simulink model "LineTrace_2025a"  (R2025a)
settings: Solver=FixedStepAuto  StartTime=0  StopTime=10  FixedStep=0.001  RelTol=1e-3
undefined symbols (not defined in the file): Rec, SDTV, Sim3dSensor
libraries: visionsinks x9, sim3dcameralib x9, sim3dlib x4, visionconversions x4
settings Model: ModifiedByFormat=The MathWorks, Inc.  Creator=The MathWorks, Inc.  LastModifiedBy=The MathWorks, Inc.
settings DataIOCC: SaveFormat=StructureWithTime
settings OptimizationCC: BlockReduction=off  BufferReuse=off
settings DebuggingCC: AlgebraicLoopMsg=none  SubsystemReferenceDiagnosticForUnitTest=warning
settings RTWCC: GPUComputeCapability=3.5

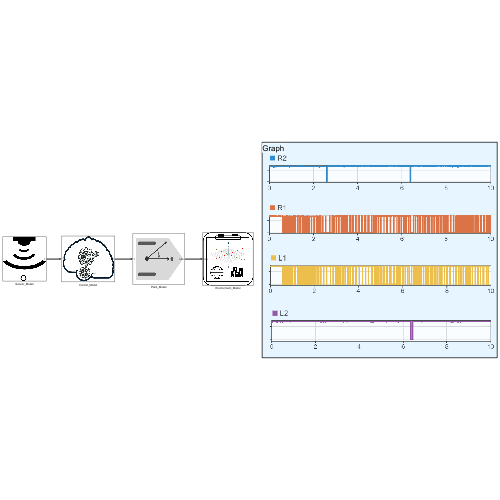
[thumbnail: Simulink's stored preview of the top-level diagram]
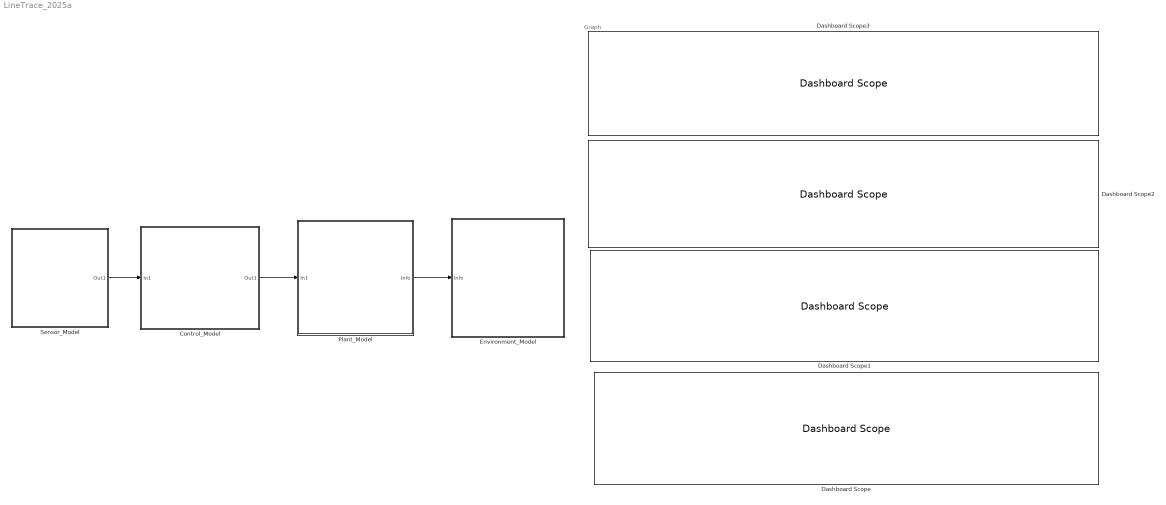
== system LineTrace_2025a ==
  note: Graph
  Control_Model : Subsystem
      mask Display: image('Control.png');
  Dashboard Scope{,1..3} (4 alike) : DashboardScope  Ymin=0  Ymax=3200  FontColor=[0.0, 0.0, 0.0]
      settings: TickLabels=T-Axis
  Environment_Model : Subsystem
      mask Display: image('Environment.png');
  Plant_Model : Subsystem
      mask Display: image('Plant.png');
  Sensor_Model : Subsystem
      mask Display: image('Sensor.png');
  wires:
  Sensor_Model/1(Out1) -> Control_Model/1(In1)
  Control_Model/1(Out1) -> Plant_Model/1(In1)
  Plant_Model/1(Info) -> Environment_Model/1(Info)

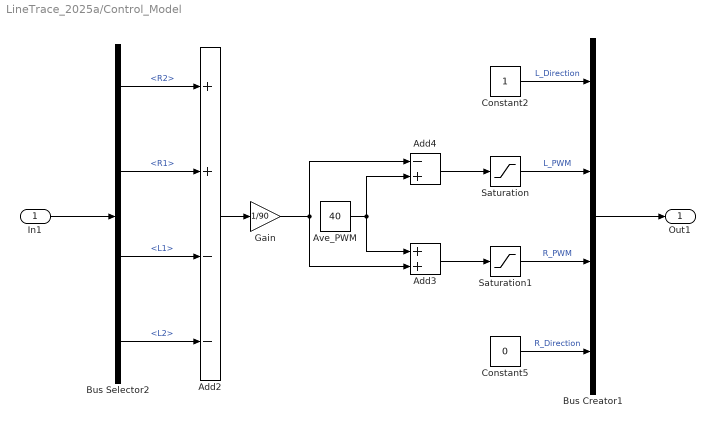
== system LineTrace_2025a/Control_Model ==
  In1 : Inport
  Add2 : Sum  Inputs=++--  OutDataTypeStr=double
  Add3 : Sum
  Add4 : Sum  Inputs=-+
  Ave_PWM : Constant  Value=40
  Bus Creator1 : BusCreator  Inputs=4
  Bus Selector2 : BusSelector  OutputSignals=R2,R1,L1,L2
  Constant2 : Constant
  Constant5 : Constant  Value=0
  Gain : Gain  Gain=1/90
  Saturation : Saturate  UpperLimit=99  LowerLimit=0
  Saturation1 : Saturate  UpperLimit=99  LowerLimit=0
  Out1 : Outport
  wires:
  Bus Selector2/2 -> Add2/2  "<R1>"
  In1/1 -> Bus Selector2/1
  Ave_PWM/1 -> Add4/2, Add3/1
  Add2/1 -> Gain/1
  Bus Selector2/4 -> Add2/4  "<L2>"
  Saturation1/1 -> Bus Creator1/3  "R_PWM"
  Saturation/1 -> Bus Creator1/2  "L_PWM"
  Constant5/1 -> Bus Creator1/4  "R_Direction"
  Add4/1 -> Saturation/1
  Add3/1 -> Saturation1/1
  Bus Selector2/1 -> Add2/1  "<R2>"
  Bus Selector2/3 -> Add2/3  "<L1>"
  Constant2/1 -> Bus Creator1/1  "L_Direction"
  Bus Creator1/1 -> Out1/1
  Gain/1 -> Add4/1, Add3/2

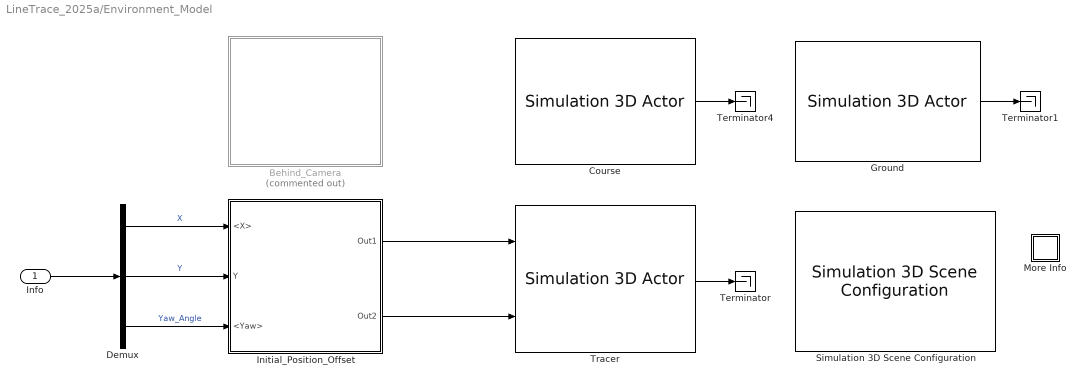
== system LineTrace_2025a/Environment_Model ==
  Info : Inport
  Behind_Camera : Subsystem  Commented=on  mask{R2_X=-0.7, R2_Y=0, R2_Z=0.2, R2_Rot_X=0, R2_Rot_Y=-pi/6, R2_Rot_Z=0}
      mask prompts: R2_X "Initial Sensor Position (X) [m]"; R2_Y "Initial Sensor Position (Y) [m]"; R2_Z "Initial Sensor Position (Z) [m]"; R2_Rot_X "Rotation Offset (X):  Roll [rad]"; R2_Rot_Y "Rotation Offset (Y): Pitch[rad]"; R2_Rot_Z "Rotation Offset (Z):  Yaw [rad]"
      mask help:
      | This block sets the initial position (X, Y, Z) and orientation (Roll, Pitch, Yaw) of the robot.
      | Simply enter the parameters to adjust accordingly.
      mask DialogControl DescTextVar Prompt: This block sets the initial position (X, Y, Z) and orientation (Roll, Pitch, Yaw) of a sensor. Simply enter the parameters to adjust accordingly. Since the sensor is facing directly downward, the initial value of Pitch is set to 90 degrees.
      mask Display: image('スクリーンショット 2025-03-12 191128.png');
  Course : sim3dlib/Simulation 3D Actor  ActorName=Course  ParentName=Scene Origin  Operation=Create at setup  InitScriptText=|  SampleTime=-1  Translation=single([0 0 0])  Rotation=single([0 0 0])  Scale=0.01*[1 1 0.01]  aMode=5  ActorTag=Course  ActorType=Sim3dActor  ID=C
      | Actor.PreciseContacts = true;
      | Actor.Physics = true;
      | Actor.Color = [0 0 0];
      | actor.Shininess = 0;
      | actor.Metallic = 0;
      settings: LibrarySourceBlock=sl3dlib/Simulation 3D/Simulation 3D Actor
  Demux : Demux  Outputs=3
  Ground : sim3dlib/Simulation 3D Actor  ActorName=Ground  ParentName=Scene Origin  Operation=Create at setup  InitScriptText=|  SampleTime=-1  Translation=single([0 0 0])  Rotation=single([0 0 0])  Scale=single([1 1 1])  aMode=5  ActorTag=Ground  ActorType=Sim3dActor  ID=C
      | Actor.createShape('plane', [3 3 0.001]);
      | Actor.PreciseContacts = true;
      | Actor.Physics = true;
      | Actor.Color = [1 1 1];
      | actor.Shininess = 0;
      | actor.Metallic = 0;
      settings: LibrarySourceBlock=sl3dlib/Simulation 3D/Simulation 3D Actor
  Initial_Position_Offset : Subsystem  mask{Offset_X=0, Offset_Y=0, Offset_Z=0, Offset_Rot_X=0, Offset_Rot_Y=0, Offset_Rot_Z=0}
      mask prompts: Offset_X "Translation Offset (X) [m]"; Offset_Y "Translation Offset (Y) [m]"; Offset_Z "Translation Offset (Z) [m]"; Offset_Rot_X "Rotation Offset (X):  Roll [rad]"; Offset_Rot_Y "Rotation Offset (Y): Pitch[rad]"; Offset_Rot_Z "Rotation Offset (Z):  Yaw [rad]"
      mask DialogControl DescTextVar Prompt: This block sets the initial position (X, Y, Z) and orientation (Roll, Pitch, Yaw) of the robot. Simply enter the parameters to adjust accordingly.
      mask Display: image('画像2.png');
  More Info : Subsystem
      settings: OpenFcn=showExample('sl3d/CreateActorSTLFileExample')
      mask Display: disp('?')
  Simulation 3D Scene Configuration : sim3dlib/Simulation 3D Scene Configuration  Priority=0  ProjectFormat=Default Scenes  SceneDesc=Empty scene  ProjectName=C:\Program Files\MATLAB\R2025a\toolbox\shared\sim3d_projects\automotive_project_windows\UE\WindowsNoEditor\VehicleSimulation.exe  ScenePath=/Game/Maps/HwStrght  EnableOpenDRIVE=off  vehTagList={'Course';'Custom';'Ground';'Scene Origin';'Tracer'}  vehTag=Custom  AttachedCameraRelativeTranslation=[0 0 0]  FreeCameraDefaultInitialTranslation=[-6, 0, 2]  AttachedCameraRelativeRotation=[0 0 0]  FreeCameraDefaultInitialRotation=[0, -15, 0]  ViewpointName=Custom  FreeCameraInitialTranslation=[0 0.6 1.5]  ViewpointTranslation=[0 0.6 1.5]  FreeCameraInitialRotation=[0 -90 90]  ViewpointRotation=[0 -90 90]  OpVisEn=off  Ts=.01  EnableWindow=on  EnableRemoteAccess=off  EnableWeather=off  SunAzimuth=90  SunAltitude=40.0  EnableGeospatialSun=off  Latitude=0  Longitude=0  Date=2023-01-01  Time=10:30:00  GeoTimeZone=-5.0  SunDaylightSaving=off  wind=1  clouds=10  EnableVolumetricClouds=off  CloudCoverage=0  CloudAltitude=6  fog=0  rain=0  RaindropsEffect=off  SnowDensity=0  EnableGeospatial=off  TilesetSource=Earth terrain  UseTrueOrigin=off  OriginHeight=200  OriginLatitude=40.744652  OriginLongitude=-73.988864  MapStyle=Aerial  AdditionalAssetIDs=[]  UseAdvancedSunSky=off  SolarTime=11  TimeZone=-5  Day=21  Month=9  Year=2022  UseDaylightSavingTime=on  DSTStartDay=10  DSTStartMonth=3  DSTEndDay=3  DSTEndMonth=11  DSTSwitchHour=2  sensorTag=MainCamera2  sensorId=2  sensorName=MainCamera2  mountLoc=Origin  offsetFlag=off  tmountOffset=[0, 0, 0]  rmountOffset=[0, 0, 0]  HorizontalResolution=1280  VerticalResolution=720  HorizontalFOV=60  mountPoint=[0 0 0]  mountOrientation=[0 0 0]  aMode=5  ID=2  GeoTrigger=Inactive  ViewNameList={'Custom'}  ViewTranslationList={'[0 0.6 1.5]'}  ViewRotationList={'[0 -90 90]'}
      settings: LibrarySourceBlock=sl3dlib/Simulation 3D/Environment/Simulation 3D Scene Configuration
  Terminator : Terminator
  Terminator1 : Terminator
  Terminator4 : Terminator
  Tracer : sim3dlib/Simulation 3D Actor  Priority=1  ActorName=Tracer  ParentName=Scene Origin  Operation=Create at setup  InitScriptText=|  SampleTime=-1  Translation=[0 0 0]  Rotation=[0 0 0]  Scale=0.01*[1 1 1]  InputsText=Tracer.Translation Tracer.Rotation  aMode=5  ActorTag=Tracer  ActorType=Sim3dActor  ID=C
      | Actor.Shadows = true;
      | Actor.Color = [0 0 0];
  wires:
  Course/1 -> Terminator4/1
  Ground/1 -> Terminator1/1
  Tracer/1 -> Terminator/1
  Initial_Position_Offset/2(Out2) -> Tracer/2
  Info/1 -> Demux/1
  Demux/1 -> Initial_Position_Offset/1(<X>)  "X"
  Demux/2 -> Initial_Position_Offset/2(Y)  "Y"
  Demux/3 -> Initial_Position_Offset/3(<Yaw>)  "Yaw_Angle"
  Initial_Position_Offset/1(Out1) -> Tracer/1

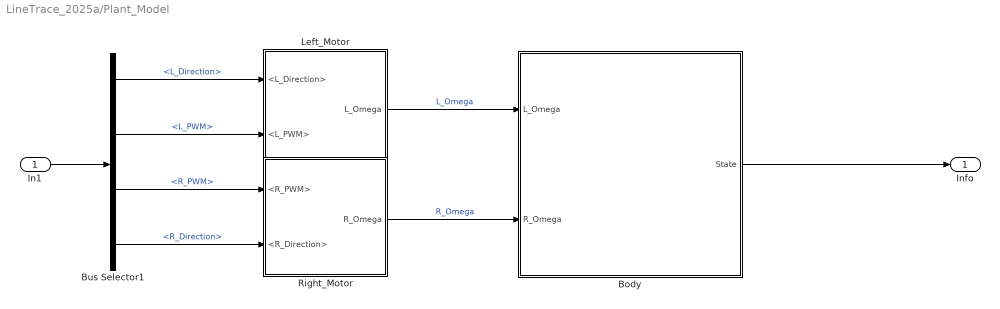
== system LineTrace_2025a/Plant_Model ==
  In1 : Inport
  Body : Subsystem  mask{Diameter_L=0.0205, Diameter_R=0.0205, Tread=0.085}
      mask prompts: Diameter_L "Left Wheel Diameter [m]"; Diameter_R "Right Wheel Diameter [m]"; Tread "Track Width [m]"
      mask DialogControl DescGroupVar Prompt: Differential Drive Kinematic Model
      mask DialogControl DescTextVar Prompt: Compute vehicle motion using a differential drive kinematic model.   The block inputs are two scalar values that depend on the value of the Vehicle inputs parameter and can either accept left and right wheel speeds, or vehicle speed and heading angular velocity. The block outputs a three-element state vector of xy-positions and vehicle heading, [x y theta], and their time derivatives, stateDot.
      mask Display: image('スクリーンショット 2025-02-13 142952.png');
  Bus Selector1 : BusSelector  OutputSignals=L_Direction,L_PWM,R_PWM,R_Direction
  Left_Motor : Subsystem
      mask Display: image('L_Motor.png');
  Right_Motor : Subsystem
      mask Display: image('R_Motor.png');
  Info : Outport
  wires:
  Body/1(State) -> Info/1
  In1/1 -> Bus Selector1/1
  Bus Selector1/1 -> Left_Motor/1(<L_Direction>)  "<L_Direction>"
  Bus Selector1/2 -> Left_Motor/2(<L_PWM>)  "<L_PWM>"
  Left_Motor/1(L_Omega) -> Body/1(L_Omega)  "L_Omega"
  Bus Selector1/3 -> Right_Motor/1(<R_PWM>)  "<R_PWM>"
  Bus Selector1/4 -> Right_Motor/2(<R_Direction>)  "<R_Direction>"
  Right_Motor/1(R_Omega) -> Body/2(R_Omega)  "R_Omega"

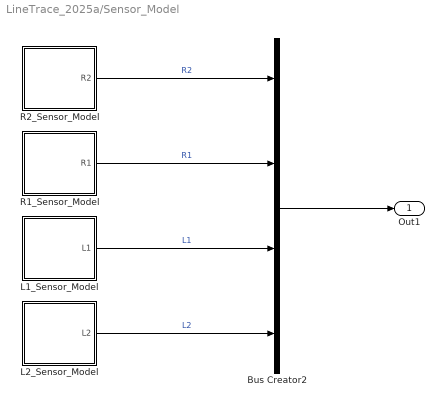
== system LineTrace_2025a/Sensor_Model ==
  Bus Creator2 : BusCreator  Inputs=4
  L1_Sensor_Model : Subsystem  mask{L1_X=0.0675, L1_Y=0.0115, L1_Z=0.0145, L1_Rot_X=0, L1_Rot_Y=-pi/2, L1_Rot_Z=0}
      mask prompts: L1_X "Initial Sensor Position (X) [m]"; L1_Y "Initial Sensor Position (Y) [m]"; L1_Z "Initial Sensor Position (Z) [m]"; L1_Rot_X "Rotation Offset (X):  Roll [rad]"; L1_Rot_Y "Rotation Offset (Y): Pitch[rad]"; L1_Rot_Z "Rotation Offset (Z):  Yaw [rad]"
      mask DialogControl DescTextVar Prompt: This block sets the initial position (X, Y, Z) and orientation (Roll, Pitch, Yaw) of a sensor. Simply enter the parameters to adjust accordingly. Since the sensor is facing directly downward, the initial value of Pitch is set to 90 degrees.
      mask Display: image('L1.png');
  L2_Sensor_Model : Subsystem  mask{L2_X=0.075, L2_Y=0.0325, L2_Z=0.0145, L2_Rot_X=0, L2_Rot_Y=-pi/2, L2_Rot_Z=0}
      mask prompts: L2_X "Initial Sensor Position (X) [m]"; L2_Y "Initial Sensor Position (Y) [m]"; L2_Z "Initial Sensor Position (Z) [m]"; L2_Rot_X "Rotation Offset (X):  Roll [rad]"; L2_Rot_Y "Rotation Offset (Y): Pitch[rad]"; L2_Rot_Z "Rotation Offset (Z):  Yaw [rad]"
      mask DialogControl DescTextVar Prompt: This block sets the initial position (X, Y, Z) and orientation (Roll, Pitch, Yaw) of a sensor. Simply enter the parameters to adjust accordingly. Since the sensor is facing directly downward, the initial value of Pitch is set to 90 degrees.
      mask Display: image('L2.png');
  R1_Sensor_Model : Subsystem  mask{R1_X=0.0675, R1_Y=-0.0115, R1_Z=0.0145, R1_Rot_X=0, R1_Rot_Y=-pi/2, R1_Rot_Z=0}
      mask prompts: R1_X "Initial Sensor Position (X) [m]"; R1_Y "Initial Sensor Position (Y) [m]"; R1_Z "Initial Sensor Position (Z) [m]"; R1_Rot_X "Rotation Offset (X):  Roll [rad]"; R1_Rot_Y "Rotation Offset (Y): Pitch[rad]"; R1_Rot_Z "Rotation Offset (Z):  Yaw [rad]"
      mask DialogControl DescTextVar Prompt: This block sets the initial position (X, Y, Z) and orientation (Roll, Pitch, Yaw) of a sensor. Simply enter the parameters to adjust accordingly. Since the sensor is facing directly downward, the initial value of Pitch is set to 90 degrees.
      mask Display: image('R1.png');
  R2_Sensor_Model : Subsystem  mask{R2_X=0.075, R2_Y=-0.0325, R2_Z=0.0145, R2_Rot_X=0, R2_Rot_Y=-pi/2, R2_Rot_Z=0}
      mask prompts: R2_X "Initial Sensor Position (X) [m]"; R2_Y "Initial Sensor Position (Y) [m]"; R2_Z "Initial Sensor Position (Z) [m]"; R2_Rot_X "Rotation Offset (X):  Roll [rad]"; R2_Rot_Y "Rotation Offset (Y): Pitch[rad]"; R2_Rot_Z "Rotation Offset (Z):  Yaw [rad]"
      mask help:
      | This block sets the initial position (X, Y, Z) and orientation (Roll, Pitch, Yaw) of the robot.
      | Simply enter the parameters to adjust accordingly.
      mask DialogControl DescTextVar Prompt: This block sets the initial position (X, Y, Z) and orientation (Roll, Pitch, Yaw) of a sensor. Simply enter the parameters to adjust accordingly. Since the sensor is facing directly downward, the initial value of Pitch is set to 90 degrees.
      mask Display: image('R2.png');
  Out1 : Outport
  wires:
  R1_Sensor_Model/1(R1) -> Bus Creator2/2  "R1"
  L1_Sensor_Model/1(L1) -> Bus Creator2/3  "L1"
  R2_Sensor_Model/1(R2) -> Bus Creator2/1  "R2"
  L2_Sensor_Model/1(L2) -> Bus Creator2/4  "L2"
  Bus Creator2/1 -> Out1/1

== system LineTrace_2025a/Environment_Model/Behind_Camera ==
  Back Camera : Subsystem
      mask Display: image('スクリーンショット 2025-03-18 120217.png');

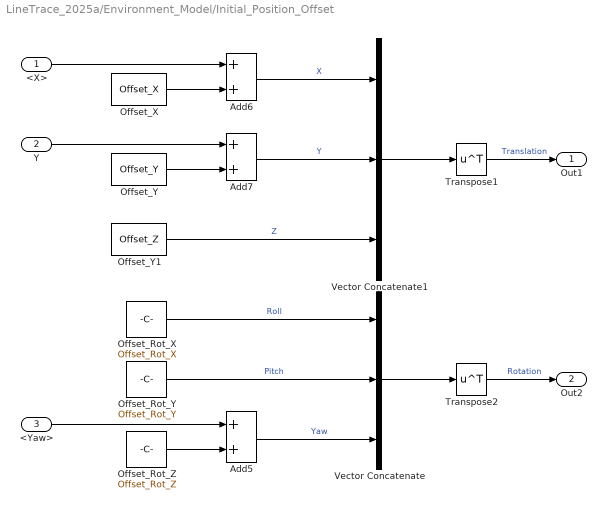
== system LineTrace_2025a/Environment_Model/Initial_Position_Offset ==
  <X> : Inport
  Y : Inport  Port=2
  <Yaw> : Inport  Port=3
  Add5 : Sum
  Add6 : Sum
  Add7 : Sum
  Offset_Rot_X : Constant  Value=Offset_Rot_X
  Offset_Rot_Y : Constant  Value=Offset_Rot_Y
  Offset_Rot_Z : Constant  Value=Offset_Rot_Z
  Offset_X : Constant  Value=Offset_X
  Offset_Y : Constant  Value=Offset_Y
  Offset_Y1 : Constant  Value=Offset_Z
  Transpose1 : Math  Operator=transpose
  Transpose2 : Math  Operator=transpose
  Vector Concatenate : Concatenate  NumInputs=3
  Vector Concatenate1 : Concatenate  NumInputs=3
  Out1 : Outport
  Out2 : Outport  Port=2
  wires:
  Add5/1 -> Vector Concatenate/3  "Yaw"
  Offset_Rot_X/1 -> Vector Concatenate/1  "Roll"
  Add7/1 -> Vector Concatenate1/2  "Y"
  Offset_Y1/1 -> Vector Concatenate1/3  "Z"
  Add6/1 -> Vector Concatenate1/1  "X"
  Offset_X/1 -> Add6/2
  Offset_Rot_Z/1 -> Add5/2
  Offset_Y/1 -> Add7/2
  Offset_Rot_Y/1 -> Vector Concatenate/2  "Pitch"
  Vector Concatenate/1 -> Transpose2/1
  Transpose1/1 -> Out1/1  "Translation"
  <Yaw>/1 -> Add5/1
  Y/1 -> Add7/1
  Vector Concatenate1/1 -> Transpose1/1
  Transpose2/1 -> Out2/1  "Rotation"
  <X>/1 -> Add6/1

== system LineTrace_2025a/Environment_Model/More Info ==

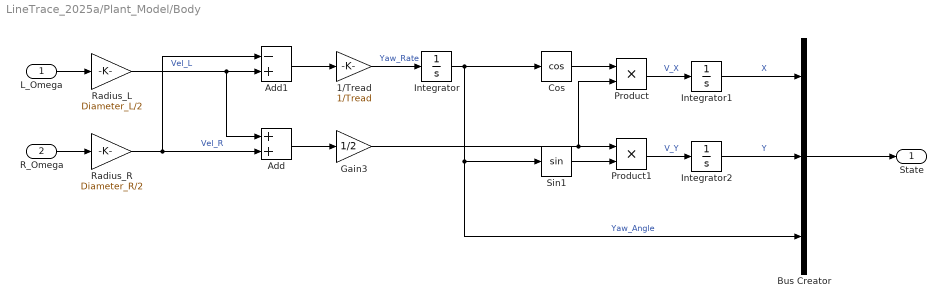
== system LineTrace_2025a/Plant_Model/Body ==
  L_Omega : Inport
  R_Omega : Inport  Port=2
  1/Tread : Gain  Gain=1/Tread
  Add : Sum
  Add1 : Sum  Inputs=-+
  Bus Creator : BusCreator  Inputs=3
  Cos : Trigonometry  Operator=cos
  Gain3 : Gain  Gain=1/2
  Integrator : Integrator
  Integrator1 : Integrator
  Integrator2 : Integrator
  Product : Product
  Product1 : Product
  Radius_L : Gain  Gain=Diameter_L/2
  Radius_R : Gain  Gain=Diameter_R/2
  Sin1 : Trigonometry
  State : Outport
  wires:
  Integrator/1 -> Bus Creator/3, Sin1/1, Cos/1  "Yaw_Angle"
  Product/1 -> Integrator1/1  "V_X"
  1/Tread/1 -> Integrator/1  "Yaw_Rate"
  Add/1 -> Gain3/1
  Sin1/1 -> Product1/2
  Cos/1 -> Product/1
  L_Omega/1 -> Radius_L/1
  Gain3/1 -> Product/2, Product1/1
  Product1/1 -> Integrator2/1  "V_Y"
  Integrator1/1 -> Bus Creator/1  "X"
  Add1/1 -> 1/Tread/1
  R_Omega/1 -> Radius_R/1
  Integrator2/1 -> Bus Creator/2  "Y"
  Bus Creator/1 -> State/1
  Radius_L/1 -> Add/1, Add1/2  "Vel_L"
  Radius_R/1 -> Add/2, Add1/1  "Vel_R"

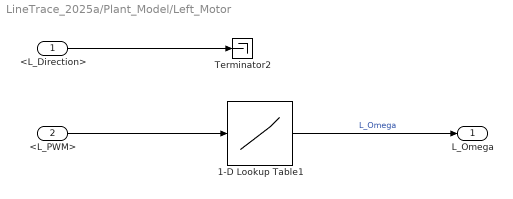
== system LineTrace_2025a/Plant_Model/Left_Motor ==
  <L_Direction> : Inport
  <L_PWM> : Inport  Port=2
  1-D Lookup Table1 : Lookup_n-D  NumberOfTableDimensions=1  BreakpointsForDimension1=[-100:20:100]  Table=tanh([-5:5])*50  InternalRulePriority=Speed  RndMeth=Simplest
  Terminator2 : Terminator
  L_Omega : Outport
  wires:
  1-D Lookup Table1/1 -> L_Omega/1  "L_Omega"
  <L_Direction>/1 -> Terminator2/1
  <L_PWM>/1 -> 1-D Lookup Table1/1

== system LineTrace_2025a/Plant_Model/Right_Motor ==
  <R_PWM> : Inport
  <R_Direction> : Inport  Port=2
  1-D Lookup Table1 : Lookup_n-D  NumberOfTableDimensions=1  BreakpointsForDimension1=[-100:20:100]  Table=tanh([-5:5])*50  InternalRulePriority=Speed  RndMeth=Simplest
  Terminator3 : Terminator
  R_Omega : Outport
  wires:
  <R_PWM>/1 -> 1-D Lookup Table1/1
  1-D Lookup Table1/1 -> R_Omega/1  "R_Omega"
  <R_Direction>/1 -> Terminator3/1

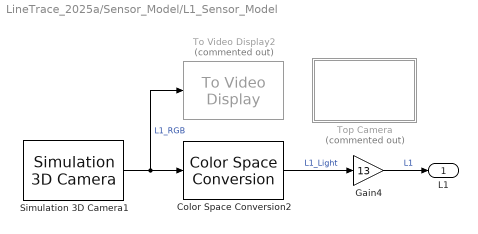
== system LineTrace_2025a/Sensor_Model/L1_Sensor_Model ==
  Color Space Conversion2 : visionconversions/Color Space  Conversion  conversion=Obsolete  conversionActive=R'G'B' to intensity  wp_str=D65  rec=Rec. 601 (SDTV)  sys=1125/60/2:1  imagePorts=One multidimensional signal
  Gain4 : Gain  Gain=13
  Simulation 3D Camera1 : sim3dcameralib/Simulation 3D Camera  Priority=1  sensorTag=Sim3dSensor$  sensorId=36  sensorName=Sim3dSensor$  vehTagList={'Course';'Ground';'Scene Origin';'Tracer'}  vehTag=Tracer  CoordinateSystem=Default  mountLoc=Origin  offsetFlag=on  tmountOffset=100*[L1_X, -L1_Y, L1_Z+0.089]  extTmount=off  rmountOffset=[L1_Rot_X L1_Rot_Y L1_Rot_Z]  extRmount=off  FocalLength=[75000 75000]  OpticalCenter=[0.5 0.5]  ImageSize=[1 1]  RadialDistortion=[0, 0]  TangentialDistortion=[0, 0]  SensorSkew=0  VisualizeFieldOfView=off  FieldOfViewRange=61  DepthOutportEnabled=off  SemanticOutportEnabled=off  TransformOutportEnabled=off  SampleTime=-1  mountPoint=[6.75 -1.15 10.35]  mountOrientation=[0 -1.5707963267949 0]  aMode=5  ID=36
      settings: LibrarySourceBlock=Simulation 3D Camera
  To Video Display2 : visionsinks/To Video Display  Commented=on  windowSizeMode=Normal  openAtMdlStart=on  fullScreen=off  videoWindowX=536805376  videoWindowY=536805376  saveWindowSize=off  videoWindowWidth=956  videoWindowHeight=1146  inputColorFormat=RGB  inputType=Obsolete  imagePorts=One multidimensional signal  OutputDevice=On-screen video monitor  dataOrg=Column-major  isWindowOpen=off
  Top Camera : Subsystem  Commented=on
      mask Display: image('スクリーンショット 2025-03-18 120217.png');
  L1 : Outport
  wires:
  Simulation 3D Camera1/1 -> To Video Display2/1, Color Space Conversion2/1  "L1_RGB"
  Gain4/1 -> L1/1  "L1"
  Color Space Conversion2/1 -> Gain4/1  "L1_Light"

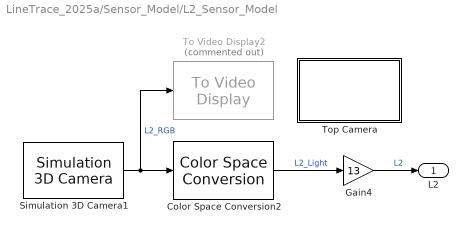
== system LineTrace_2025a/Sensor_Model/L2_Sensor_Model ==
  Color Space Conversion2 : visionconversions/Color Space  Conversion  conversion=Obsolete  conversionActive=R'G'B' to intensity  wp_str=D65  rec=Rec. 601 (SDTV)  sys=1125/60/2:1  imagePorts=One multidimensional signal
  Gain4 : Gain  Gain=13
  Simulation 3D Camera1 : sim3dcameralib/Simulation 3D Camera  Priority=1  sensorTag=Sim3dSensor&  sensorId=38  sensorName=Sim3dSensor&  vehTagList={'Course';'Ground';'Scene Origin';'Tracer'}  vehTag=Tracer  CoordinateSystem=Default  mountLoc=Origin  offsetFlag=on  tmountOffset=100*[L2_X, -L2_Y, L2_Z+0.089]  extTmount=off  rmountOffset=[L2_Rot_X L2_Rot_Y L2_Rot_Z]  extRmount=off  FocalLength=[75000 75000]  OpticalCenter=[0.5 0.5]  ImageSize=[1 1]  RadialDistortion=[0, 0]  TangentialDistortion=[0, 0]  SensorSkew=0  VisualizeFieldOfView=off  FieldOfViewRange=61  DepthOutportEnabled=off  SemanticOutportEnabled=off  TransformOutportEnabled=off  SampleTime=-1  mountPoint=[7.5 -3.25 10.35]  mountOrientation=[0 -1.5707963267949 0]  aMode=5  ID=38
      settings: LibrarySourceBlock=Simulation 3D Camera
  To Video Display2 : visionsinks/To Video Display  Commented=on  windowSizeMode=Normal  openAtMdlStart=on  fullScreen=off  videoWindowX=536805376  videoWindowY=536805376  saveWindowSize=off  videoWindowWidth=956  videoWindowHeight=1146  inputColorFormat=RGB  inputType=Obsolete  imagePorts=One multidimensional signal  OutputDevice=On-screen video monitor  dataOrg=Column-major  isWindowOpen=off
  Top Camera : Subsystem
      mask Display: image('スクリーンショット 2025-03-18 120217.png');
  L2 : Outport
  wires:
  Color Space Conversion2/1 -> Gain4/1  "L2_Light"
  Simulation 3D Camera1/1 -> To Video Display2/1, Color Space Conversion2/1  "L2_RGB"
  Gain4/1 -> L2/1  "L2"

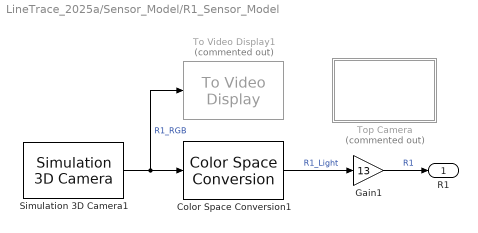
== system LineTrace_2025a/Sensor_Model/R1_Sensor_Model ==
  Color Space Conversion1 : visionconversions/Color Space  Conversion  conversion=Obsolete  conversionActive=R'G'B' to intensity  wp_str=D65  rec=Rec. 601 (SDTV)  sys=1125/60/2:1  imagePorts=One multidimensional signal
  Gain1 : Gain  Gain=13
  Simulation 3D Camera1 : sim3dcameralib/Simulation 3D Camera  Priority=1  sensorTag="Sim3dSensor\""  sensorId=34  sensorName="Sim3dSensor\""  vehTagList={'Course';'Ground';'Scene Origin';'Tracer'}  vehTag=Tracer  CoordinateSystem=Default  mountLoc=Origin  offsetFlag=on  tmountOffset=100*[R1_X, -R1_Y, R1_Z+0.089]  extTmount=off  rmountOffset=[R1_Rot_X R1_Rot_Y R1_Rot_Z]  extRmount=off  FocalLength=[75000 75000]  OpticalCenter=[0.5 0.5]  ImageSize=[1 1]  RadialDistortion=[0, 0]  TangentialDistortion=[0, 0]  SensorSkew=0  VisualizeFieldOfView=off  FieldOfViewRange=61  DepthOutportEnabled=off  SemanticOutportEnabled=off  TransformOutportEnabled=off  SampleTime=-1  mountPoint=[6.75 1.15 10.35]  mountOrientation=[0 -1.5707963267949 0]  aMode=5  ID=34
      settings: LibrarySourceBlock=Simulation 3D Camera
  To Video Display1 : visionsinks/To Video Display  Commented=on  windowSizeMode=Normal  openAtMdlStart=on  fullScreen=off  videoWindowX=536805376  videoWindowY=536805376  saveWindowSize=off  videoWindowWidth=956  videoWindowHeight=1146  inputColorFormat=RGB  inputType=Obsolete  imagePorts=One multidimensional signal  OutputDevice=On-screen video monitor  dataOrg=Column-major  isWindowOpen=off
  Top Camera : Subsystem  Commented=on
      mask Display: image('スクリーンショット 2025-03-18 120217.png');
  R1 : Outport
  wires:
  Color Space Conversion1/1 -> Gain1/1  "R1_Light"
  Gain1/1 -> R1/1  "R1"
  Simulation 3D Camera1/1 -> Color Space Conversion1/1, To Video Display1/1  "R1_RGB"

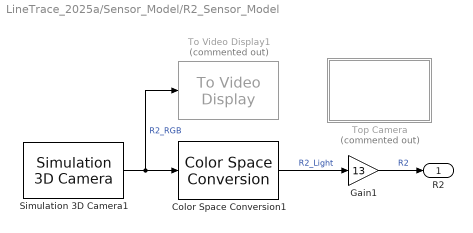
== system LineTrace_2025a/Sensor_Model/R2_Sensor_Model ==
  Color Space Conversion1 : visionconversions/Color Space  Conversion  conversion=Obsolete  conversionActive=R'G'B' to intensity  wp_str=D65  rec=Rec. 601 (SDTV)  sys=1125/60/2:1  imagePorts=One multidimensional signal
  Gain1 : Gain  Gain=13
  Simulation 3D Camera1 : sim3dcameralib/Simulation 3D Camera  Priority=1  sensorTag=Sim3dSensor  sensorId=32  sensorName=Sim3dSensor  vehTagList={'Course';'Ground';'Scene Origin';'Tracer'}  vehTag=Tracer  CoordinateSystem=Default  mountLoc=Origin  offsetFlag=on  tmountOffset=100*[R2_X, -R2_Y, R2_Z+0.089]  extTmount=off  rmountOffset=[R2_Rot_X R2_Rot_Y R2_Rot_Z]  extRmount=off  FocalLength=[75000 75000]  OpticalCenter=[0.5 0.5]  ImageSize=[1 1]  RadialDistortion=[0, 0]  TangentialDistortion=[0, 0]  SensorSkew=0  VisualizeFieldOfView=off  FieldOfViewRange=61  DepthOutportEnabled=off  SemanticOutportEnabled=off  TransformOutportEnabled=off  SampleTime=-1  mountPoint=[7.5 3.25 10.35]  mountOrientation=[0 -1.5707963267949 0]  aMode=5  ID=32
      settings: LibrarySourceBlock=Simulation 3D Camera
  To Video Display1 : visionsinks/To Video Display  Commented=on  windowSizeMode=Normal  openAtMdlStart=on  fullScreen=off  videoWindowX=536805376  videoWindowY=536805376  saveWindowSize=off  videoWindowWidth=956  videoWindowHeight=1146  inputColorFormat=RGB  inputType=Obsolete  imagePorts=One multidimensional signal  OutputDevice=On-screen video monitor  dataOrg=Column-major  isWindowOpen=off
  Top Camera : Subsystem  Commented=on
      mask Display: image('スクリーンショット 2025-03-18 120217.png');
  R2 : Outport
  wires:
  Gain1/1 -> R2/1  "R2"
  Color Space Conversion1/1 -> Gain1/1  "R2_Light"
  Simulation 3D Camera1/1 -> Color Space Conversion1/1, To Video Display1/1  "R2_RGB"

== system LineTrace_2025a/Environment_Model/Behind_Camera/Back Camera ==
  Behind_Camera : visionsinks/To Video Display  windowSizeMode=Normal  openAtMdlStart=on  fullScreen=off  videoWindowX=536805376  videoWindowY=536805376  saveWindowSize=off  videoWindowWidth=1920  videoWindowHeight=1076  inputColorFormat=RGB  inputType=Obsolete  imagePorts=One multidimensional signal  OutputDevice=On-screen video monitor  dataOrg=Column-major  isWindowOpen=off
  Simulation 3D Camera : sim3dcameralib/Simulation 3D Camera  Priority=1  sensorTag=Sim3dSensor(  sensorId=40  sensorName=Sim3dSensor(  vehTagList={'Course';'Ground';'Scene Origin';'Tracer'}  vehTag=Tracer  CoordinateSystem=Default  mountLoc=Origin  offsetFlag=on  tmountOffset=100*[R2_X, -R2_Y, R2_Z+0.3]  extTmount=off  rmountOffset=[R2_Rot_X R2_Rot_Y R2_Rot_Z]  extRmount=off  FocalLength=[2000 2000]  OpticalCenter=[500 500]  ImageSize=[1000 1000]  RadialDistortion=[0, 0]  TangentialDistortion=[0, 0]  SensorSkew=0  VisualizeFieldOfView=off  FieldOfViewRange=61  DepthOutportEnabled=off  SemanticOutportEnabled=off  TransformOutportEnabled=off  SampleTime=-1  mountPoint=[-70 0 50]  mountOrientation=[0 -0.523598775598299 0]  aMode=5  ID=40
      settings: LibrarySourceBlock=Simulation 3D Camera
  wires:
  Simulation 3D Camera/1 -> Behind_Camera/1

== system LineTrace_2025a/Sensor_Model/L1_Sensor_Model/Top Camera ==
  L1_Camera : visionsinks/To Video Display  windowSizeMode=Normal  openAtMdlStart=on  fullScreen=off  videoWindowX=536805376  videoWindowY=536805376  saveWindowSize=off  videoWindowWidth=1894  videoWindowHeight=1134  inputColorFormat=RGB  inputType=Obsolete  imagePorts=One multidimensional signal  OutputDevice=On-screen video monitor  dataOrg=Column-major  isWindowOpen=off
  Simulation 3D Camera : sim3dcameralib/Simulation 3D Camera  Priority=1  sensorTag=Sim3dSensor%  sensorId=37  sensorName=Sim3dSensor%  vehTagList={'Course';'Ground';'Scene Origin';'Tracer'}  vehTag=Tracer  CoordinateSystem=Default  mountLoc=Origin  offsetFlag=on  tmountOffset=100*[L1_X, -L1_Y, L1_Z+0.3]  extTmount=off  rmountOffset=[L1_Rot_X L1_Rot_Y L1_Rot_Z]  extRmount=off  FocalLength=[500 500]  OpticalCenter=[100 100]  ImageSize=[200 200]  RadialDistortion=[0, 0]  TangentialDistortion=[0, 0]  SensorSkew=0  VisualizeFieldOfView=off  FieldOfViewRange=61  DepthOutportEnabled=off  SemanticOutportEnabled=off  TransformOutportEnabled=off  SampleTime=-1  mountPoint=[6.75 1.15 31.45]  mountOrientation=[0 -1.5707963267949 0]  aMode=5  ID=37
      settings: LibrarySourceBlock=Simulation 3D Camera
  wires:
  Simulation 3D Camera/1 -> L1_Camera/1

== system LineTrace_2025a/Sensor_Model/L2_Sensor_Model/Top Camera ==
  L2_Camera : visionsinks/To Video Display  windowSizeMode=Normal  openAtMdlStart=on  fullScreen=off  videoWindowX=536805376  videoWindowY=536805376  saveWindowSize=off  videoWindowWidth=1894  videoWindowHeight=1134  inputColorFormat=RGB  inputType=Obsolete  imagePorts=One multidimensional signal  OutputDevice=On-screen video monitor  dataOrg=Column-major  isWindowOpen=off
  Simulation 3D Camera : sim3dcameralib/Simulation 3D Camera  Priority=1  sensorTag=Sim3dSensor'  sensorId=39  sensorName=Sim3dSensor'  vehTagList={'Course';'Ground';'Scene Origin';'Tracer'}  vehTag=Tracer  CoordinateSystem=Default  mountLoc=Origin  offsetFlag=on  tmountOffset=100*[L2_X, -L2_Y, L2_Z+0.3]  extTmount=off  rmountOffset=[L2_Rot_X L2_Rot_Y L2_Rot_Z]  extRmount=off  FocalLength=[500 500]  OpticalCenter=[100 100]  ImageSize=[200 200]  RadialDistortion=[0, 0]  TangentialDistortion=[0, 0]  SensorSkew=0  VisualizeFieldOfView=off  FieldOfViewRange=61  DepthOutportEnabled=off  SemanticOutportEnabled=off  TransformOutportEnabled=off  SampleTime=-1  mountPoint=[7.5 -3.25 31.45]  mountOrientation=[0 -1.5707963267949 0]  aMode=5  ID=39
      settings: LibrarySourceBlock=Simulation 3D Camera
  wires:
  Simulation 3D Camera/1 -> L2_Camera/1

== system LineTrace_2025a/Sensor_Model/R1_Sensor_Model/Top Camera ==
  R1_Camera : visionsinks/To Video Display  windowSizeMode=Normal  openAtMdlStart=on  fullScreen=off  videoWindowX=536805376  videoWindowY=536805376  saveWindowSize=off  videoWindowWidth=1894  videoWindowHeight=1134  inputColorFormat=RGB  inputType=Obsolete  imagePorts=One multidimensional signal  OutputDevice=On-screen video monitor  dataOrg=Column-major  isWindowOpen=off
  Simulation 3D Camera : sim3dcameralib/Simulation 3D Camera  Priority=1  sensorTag=Sim3dSensor#  sensorId=35  sensorName=Sim3dSensor#  vehTagList={'Course';'Ground';'Scene Origin';'Tracer'}  vehTag=Tracer  CoordinateSystem=Default  mountLoc=Origin  offsetFlag=on  tmountOffset=100*[R1_X, -R1_Y, R1_Z+0.3]  extTmount=off  rmountOffset=[R1_Rot_X R1_Rot_Y R1_Rot_Z]  extRmount=off  FocalLength=[500 500]  OpticalCenter=[100 100]  ImageSize=[200 200]  RadialDistortion=[0, 0]  TangentialDistortion=[0, 0]  SensorSkew=0  VisualizeFieldOfView=off  FieldOfViewRange=61  DepthOutportEnabled=off  SemanticOutportEnabled=off  TransformOutportEnabled=off  SampleTime=-1  mountPoint=[6.75 -1.15 31.45]  mountOrientation=[0 -1.5707963267949 0]  aMode=5  ID=35
      settings: LibrarySourceBlock=Simulation 3D Camera
  wires:
  Simulation 3D Camera/1 -> R1_Camera/1

== system LineTrace_2025a/Sensor_Model/R2_Sensor_Model/Top Camera ==
  R2_Camera : visionsinks/To Video Display  windowSizeMode=Normal  openAtMdlStart=on  fullScreen=off  videoWindowX=536805376  videoWindowY=536805376  saveWindowSize=off  videoWindowWidth=1894  videoWindowHeight=1134  inputColorFormat=RGB  inputType=Obsolete  imagePorts=One multidimensional signal  OutputDevice=On-screen video monitor  dataOrg=Column-major  isWindowOpen=off
  Simulation 3D Camera : sim3dcameralib/Simulation 3D Camera  Priority=1  sensorTag=Sim3dSensor!  sensorId=33  sensorName=Sim3dSensor!  vehTagList={'Course';'Ground';'Scene Origin';'Tracer'}  vehTag=Tracer  CoordinateSystem=Default  mountLoc=Origin  offsetFlag=on  tmountOffset=100*[R2_X, -R2_Y, R2_Z+0.3]  extTmount=off  rmountOffset=[R2_Rot_X R2_Rot_Y R2_Rot_Z]  extRmount=off  FocalLength=[500 500]  OpticalCenter=[100 100]  ImageSize=[200 200]  RadialDistortion=[0, 0]  TangentialDistortion=[0, 0]  SensorSkew=0  VisualizeFieldOfView=off  FieldOfViewRange=61  DepthOutportEnabled=off  SemanticOutportEnabled=off  TransformOutportEnabled=off  SampleTime=-1  mountPoint=[7.5 3.25 31.45]  mountOrientation=[0 -1.5707963267949 0]  aMode=5  ID=33
      settings: LibrarySourceBlock=Simulation 3D Camera
  wires:
  Simulation 3D Camera/1 -> R2_Camera/1
